simulink model "Ofline_LQ"  (R2022b)
settings: Solver=VariableStepAuto  StartTime=0.0  StopTime=30  RelTol=1e-3
undefined symbols (not defined in the file): A, B, C, D, K_lqeta, K_lqx, voltage_max
settings Model: Creator=utente  LastModifiedBy=utente
settings SolverCC: AlgebraicLoopSolver=TrustRegion
settings DebuggingCC: UnconnectedInputMsg=warning  UnconnectedOutputMsg=warning  UnconnectedLineMsg=warning  SFMachineParentedDataDiag=warning
settings ModelReferenceCC: EnableRefExpFcnMdlSchedulingChecks=on

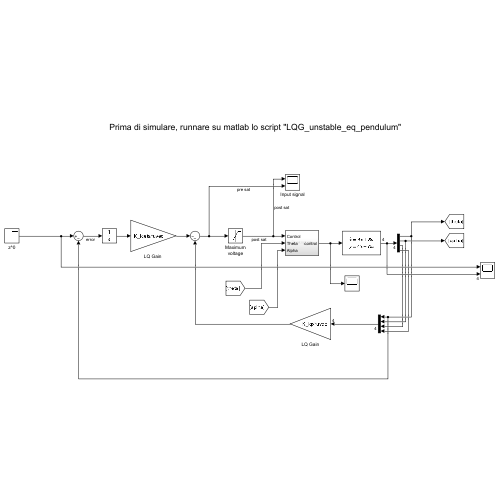
[thumbnail: Simulink's stored preview of the top-level diagram]
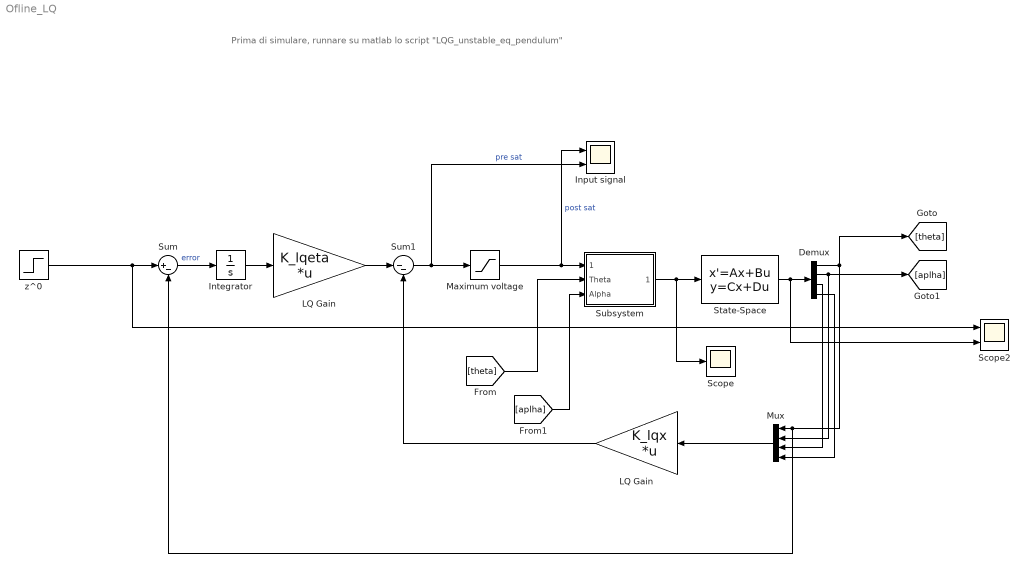
== system Ofline_LQ ==
  note: Prima di simulare, runnare su matlab lo script "LQG_unstable_eq_pendulum"
  Demux : Demux
  Input signal : Scope  NumInputPorts=2
  Integrator : Integrator
  LQ Gain : Gain  Gain=K_lqx  Multiplication=Matrix(K*u) (u vector)
  "LQ Gain " : Gain  Gain=K_lqeta  Multiplication=Matrix(K*u) (u vector)
  Maximum voltage : Saturate  UpperLimit=voltage_max  LowerLimit=-voltage_max
  Mux : Mux
  Scope : Scope
  Scope2 : Scope  NumInputPorts=2
  State-Space : StateSpace  A=A  B=B  C=C  D=D  InitialCondition=[0 0 0 0]
  Subsystem : Subsystem
  Sum : Sum  Inputs=|+-
  Sum1 : Sum  Inputs=|--
  z^0 : Step  Time=5  After=0.3  SampleTime=0
  wires:
  Maximum voltage/1 -> Input signal/1, Subsystem/1(Control)  "post sat"
  Sum/1 -> Integrator/1  "error"
  [theta] -> Subsystem/2(Theta)
  [aplha] -> Subsystem/3(Alpha)
  Subsystem/1(control) -> Scope/1, State-Space/1
  z^0/1 -> Scope2/1, Sum/1
  Integrator/1 -> "LQ Gain "/1
  "LQ Gain "/1 -> Sum1/1
  Sum1/1 -> Input signal/2, Maximum voltage/1  "pre sat"
  State-Space/1 -> Scope2/2, Demux/1
  Demux/1 -> [theta], Sum/2, Mux/1
  Demux/2 -> Mux/2, [aplha]
  Demux/3 -> Mux/3
  Demux/4 -> Mux/4
  Mux/1 -> LQ Gain/1
  LQ Gain/1 -> Sum1/2

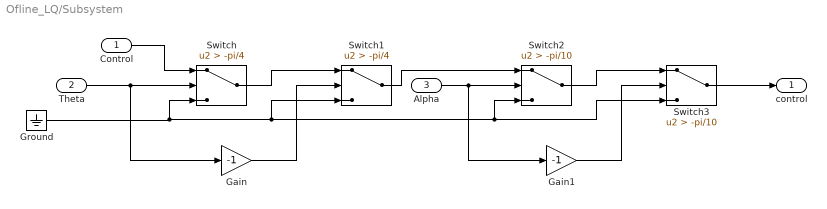
== system Ofline_LQ/Subsystem ==
  Control : Inport
  Theta : Inport  Port=2
  Alpha : Inport  Port=3
  Gain : Gain  Gain=-1
  Gain1 : Gain  Gain=-1
  Ground : Ground
  Switch : Switch  Criteria=u2 > Threshold  Threshold=-pi/4  SaturateOnIntegerOverflow=off  InputSameDT=off
  Switch1 : Switch  Criteria=u2 > Threshold  Threshold=-pi/4  SaturateOnIntegerOverflow=off  InputSameDT=off
  Switch2 : Switch  Criteria=u2 > Threshold  Threshold=-pi/10  SaturateOnIntegerOverflow=off  InputSameDT=off
  Switch3 : Switch  Criteria=u2 > Threshold  Threshold=-pi/10  SaturateOnIntegerOverflow=off  InputSameDT=off
  control : Outport
  wires:
  Gain/1 -> Switch1/2
  Theta/1 -> Gain/1, Switch/2
  Control/1 -> Switch/1
  Switch/1 -> Switch1/1
  Gain1/1 -> Switch3/2
  Switch1/1 -> Switch2/1
  Ground/1 -> Switch3/3, Switch2/3, Switch1/3, Switch/3
  Switch2/1 -> Switch3/1
  Alpha/1 -> Switch2/2, Gain1/1
  Switch3/1 -> control/1
